simulink model "inversor_1"  (R2021b)
settings: Solver=FixedStepDiscrete  StartTime=0.0  StopTime=7  FixedStep=Tint  MaxStep=1e-6  RelTol=1e-6
InitFcn:
  | run init_fcn.m;
values from neighbouring files (symbols this model uses):
  C_load = 5e-2    (= 0.05)    [init_fcn.m]    (also in init_fcn_2.m)
  L_s = 5e-3    (= 0.005)    [init_fcn.m]    (also in init_fcn_2.m)
  R_load = 10    [init_fcn.m]    (also in init_fcn_2.m)
  shift = (180/2)/360 * Ts    (= 0.000125)    [init_fcn.m]    (also in init_fcn_2.m = 8.33333333333e-05)
  Tint = 1e-6    (= 1e-06)    [init_fcn.m]    (also in init_fcn_2.m)
  Ts = 1/2000    (= 0.0005)    [init_fcn.m]    (also in init_fcn_2.m)
  V_source = 230 * sqrt(2)    [init_fcn.m]    (also in init_fcn_2.m)
libraries: spsIGBTDiodeLib x8, spsVoltageMeasurementLib x6, simulink x3, spsSeriesRLCBranchLib x3, spsParallelRLCBranchLib x2, spsACVoltageSourceLib x1, spsCurrentMeasurementLib x1, spspowerguiLib x1
settings Model: Creator=david  LastModifiedBy=david

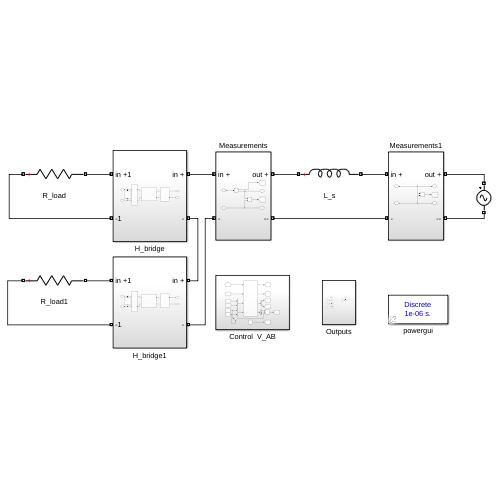
[thumbnail: Simulink's stored preview of the top-level diagram]
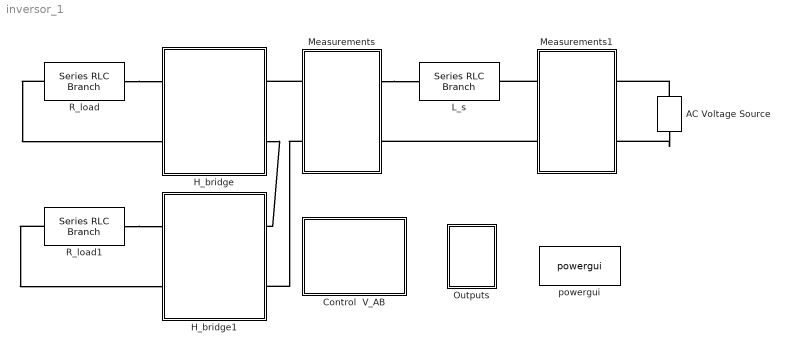
== system inversor_1 ==
  AC Voltage Source : spsACVoltageSourceLib/AC Voltage Source  Amplitude=V_source  Phase=0  Frequency=50  SampleTime=0  Measurements=None  BusType=swing  Pref=10e3  Qref=0  Qmin=-inf  Qmax=+inf
  Control  V_AB : Subsystem
  H_bridge : Subsystem
  H_bridge1 : Subsystem
  L_s : spsSeriesRLCBranchLib/Series RLC Branch  LConnTagsString=__new0  RConnTagsString=__new0  BranchType=L  Resistance=1  Inductance=L_s  SetiL0=off  InitialCurrent=0  Capacitance=1e-6  Setx0=off  InitialVoltage=0  Measurements=None
  Measurements : Subsystem
  Measurements1 : Subsystem
  Outputs : Subsystem
  R_load : spsSeriesRLCBranchLib/Series RLC Branch  LConnTagsString=__new0  RConnTagsString=__new0  BranchType=R  Resistance=R_load  Inductance=L_s  SetiL0=off  InitialCurrent=0  Capacitance=1e-6  Setx0=off  InitialVoltage=0  Measurements=None
  R_load1 : spsSeriesRLCBranchLib/Series RLC Branch  LConnTagsString=__new0  RConnTagsString=__new0  BranchType=R  Resistance=R_load  Inductance=L_s  SetiL0=off  InitialCurrent=0  Capacitance=1e-6  Setx0=off  InitialVoltage=0  Measurements=None
  powergui : spspowerguiLib/powergui  Priority=1  SimulationMode=Discrete  SampleTime=Tint  frequency=60  Iterations=50  frequencyindice=50  Pbase=100e6  ErrMax=1e-4  UnitsV=kV  UnitsW=MW  buscounter=0  FunctionMessages=off  echomessages=off  EnableUseOfTLC=off  CurrentSourceSwitches=off  DisableSnubberDevices=off  DisableRonSwitches=off  DisableVfSwitches=off  DisplayEquations=off  AutomaticDiscreteSolvers=off  SolverType=Tustin/Backward Euler (TBE)  Interpol=off  ExternalGateDelay=off  methode=off  Ts=100  x0status=blocks  SPID=on  SwTol=0  HookPort=off  NonlinearTolerance=1e-4  nMaxIteration=100  ContinueOnMaxIteration=off  RestoreLinks=warning  ResistiveCurrentMeasurement=off  Frange=[0:2:500]  Ylog=off  Xlog=on  ShowGrid=off  save=off  variable=ZData  structure=0  ZoomFFT=off  StartTime=0.0  cycles=1  DisplayStyle=1  fundamental=60  FreqAxis=off  MaxFrequency=1000  frequencyindicesteady=1  RmsSteady=1  display=off
  connections:
  R_load/LConn1 -- H_bridge/LConn2
  R_load/RConn1 -- H_bridge/LConn1
  Measurements/LConn1 -- H_bridge/RConn1
  Measurements/RConn1 -- L_s/LConn1
  Measurements1/LConn2 -- Measurements/RConn2
  Measurements1/LConn1 -- L_s/RConn1
  AC Voltage Source/RConn1 -- Measurements1/RConn1
  AC Voltage Source/LConn1 -- Measurements1/RConn2
  Measurements/LConn2 -- H_bridge1/RConn2
  R_load1/RConn1 -- H_bridge1/LConn1
  R_load1/LConn1 -- H_bridge1/LConn2
  H_bridge/RConn2 -- H_bridge1/RConn1

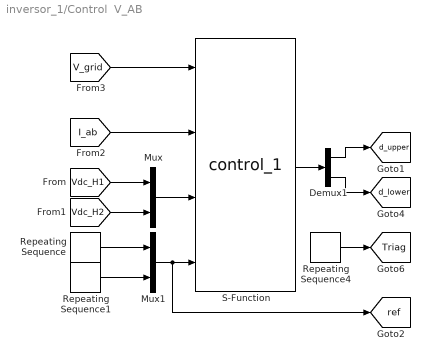
== system inversor_1/Control  V_AB ==
  Demux1 : Demux  Outputs=2
  Mux : Mux  Inputs=2
  Mux1 : Mux  Inputs=2
  Repeating Sequence : simulink/Sources/Repeating Sequence  rep_seq_t=[0 2 3 4 5 7]  rep_seq_y=[200 200 250 250 200 180]
  Repeating Sequence1 : simulink/Sources/Repeating Sequence  rep_seq_t=[0 2 3 4 5 7]  rep_seq_y=[200 200 150 150 230 230]
  Repeating Sequence4 : simulink/Sources/Repeating Sequence  rep_seq_t=[0 Ts/2 Ts]  rep_seq_y=[-1 1 -1]
  S-Function : S-Function  FunctionName=control_1  SFunctionDeploymentMode=off  EnableBusSupport=off
  tag scope: Triag=global, d_lower=global, d_upper=global, ref=global
  wires:
  Mux/1 -> S-Function/3
  [Vdc_H1] -> Mux/1
  [I_ab] -> S-Function/2
  [V_grid] -> S-Function/1
  Repeating Sequence/1 -> Mux1/1
  Repeating Sequence1/1 -> Mux1/2
  [Vdc_H2] -> Mux/2
  S-Function/1 -> Demux1/1
  Demux1/1 -> [d_upper]
  Demux1/2 -> [d_lower]
  Repeating Sequence4/1 -> [Triag]
  Mux1/1 -> [ref], S-Function/4

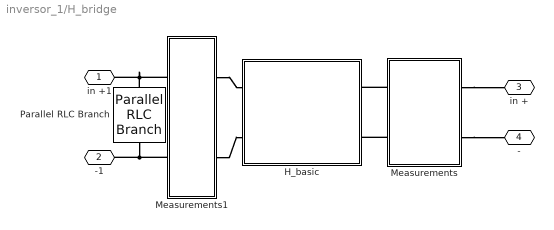
== system inversor_1/H_bridge ==
  H_basic : Subsystem
  Measurements : Subsystem
  Measurements1 : Subsystem
  Parallel RLC Branch : spsParallelRLCBranchLib/Parallel RLC Branch  LConnTagsString=a  RConnTagsString=__new0  BranchType=C  Resistance=1  Inductance=1e-3  SetiL0=off  InitialCurrent=0  Capacitance=C_load  Setx0=on  InitialVoltage=C_init_v  Measurements=None
  in +1 : PMIOPort  Side=Left
  -1 : PMIOPort  Port=2  Side=Left
  in + : PMIOPort  Port=3  Side=Right
  - : PMIOPort  Port=4  Side=Right
  connections:
  Measurements1/RConn1 -- H_basic/LConn1
  Measurements/LConn1 -- in +/RConn1
  Measurements1/RConn2 -- H_basic/LConn2
  Measurements1/LConn1 -- Parallel RLC Branch/LConn1 -- in +1/RConn1
  Measurements1/LConn2 -- Parallel RLC Branch/RConn1 -- -1/RConn1
  Measurements/RConn2 -- H_basic/RConn2
  Measurements/LConn2 -- -/RConn1
  Measurements/RConn1 -- H_basic/RConn1

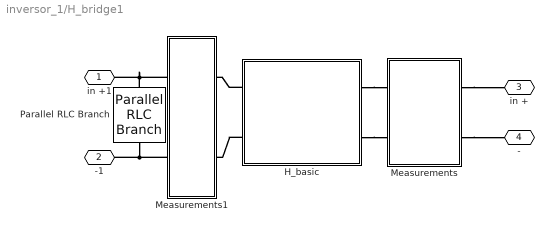
== system inversor_1/H_bridge1 ==
  H_basic : Subsystem
  Measurements : Subsystem
  Measurements1 : Subsystem
  Parallel RLC Branch : spsParallelRLCBranchLib/Parallel RLC Branch  LConnTagsString=a  RConnTagsString=__new0  BranchType=C  Resistance=1  Inductance=1e-3  SetiL0=off  InitialCurrent=0  Capacitance=C_load  Setx0=on  InitialVoltage=C_init_v  Measurements=None
  in +1 : PMIOPort  Side=Left
  -1 : PMIOPort  Port=2  Side=Left
  in + : PMIOPort  Port=3  Side=Right
  - : PMIOPort  Port=4  Side=Right
  connections:
  H_basic/LConn1 -- Measurements1/RConn1
  Measurements/LConn1 -- in +/RConn1
  H_basic/LConn2 -- Measurements1/RConn2
  Measurements1/LConn1 -- Parallel RLC Branch/LConn1 -- in +1/RConn1
  Measurements1/LConn2 -- Parallel RLC Branch/RConn1 -- -1/RConn1
  H_basic/RConn2 -- Measurements/RConn2
  Measurements/LConn2 -- -/RConn1
  H_basic/RConn1 -- Measurements/RConn1

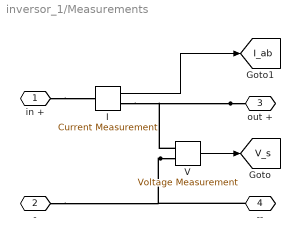
== system inversor_1/Measurements ==
  I : spsCurrentMeasurementLib/Current Measurement  PhasorSimulation=off  OutputType=Complex  PSBequivalent=0
  V : spsVoltageMeasurementLib/Voltage Measurement  PhasorSimulation=off  OutputType=Complex  PSBequivalent=0
  in + : PMIOPort  Side=Left
  - : PMIOPort  Port=2  Side=Left
  out + : PMIOPort  Port=3  Side=Right
  -- : PMIOPort  Port=4  Side=Right
  tag scope: I_ab=global, V_s=global
  wires:
  V/1 -> [V_s]
  I/1 -> [I_ab]
  connections:
  V/LConn2 -- --/RConn1 -- -/RConn1
  out +/RConn1 -- V/LConn1 -- I/RConn1
  in +/RConn1 -- I/LConn1

== system inversor_1/Measurements1 ==
  V : spsVoltageMeasurementLib/Voltage Measurement  PhasorSimulation=off  OutputType=Complex  PSBequivalent=0
  in + : PMIOPort  Side=Left
  - : PMIOPort  Port=2  Side=Left
  out + : PMIOPort  Port=3  Side=Right
  -- : PMIOPort  Port=4  Side=Right
  tag scope: V_grid=global
  wires:
  V/1 -> [V_grid]
  connections:
  V/LConn2 -- --/RConn1 -- -/RConn1
  out +/RConn1 -- in +/RConn1 -- V/LConn1

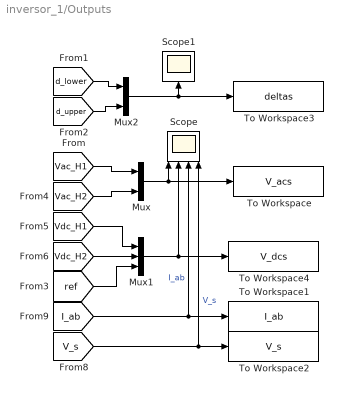
== system inversor_1/Outputs ==
  Mux : Mux  Inputs=2
  Mux1 : Mux  Inputs=3
  Mux2 : Mux  Inputs=2
  Scope : Scope  NumInputPorts=4
  Scope1 : Scope
  To Workspace : ToWorkspace  VariableName=V_acs  SaveFormat=Structure With Time  SampleTime=-1
  To Workspace1 : ToWorkspace  VariableName=I_ab  SaveFormat=Structure With Time  SampleTime=-1
  To Workspace2 : ToWorkspace  VariableName=V_s  SaveFormat=Structure With Time  SampleTime=-1
  To Workspace3 : ToWorkspace  VariableName=deltas  SaveFormat=Structure With Time  SampleTime=-1
  To Workspace4 : ToWorkspace  VariableName=V_dcs  SaveFormat=Structure With Time  SampleTime=-1
  wires:
  Mux/1 -> Scope/1, To Workspace/1
  [Vac_H1] -> Mux/1
  [Vac_H2] -> Mux/2
  Mux1/1 -> Scope/2, To Workspace4/1
  [V_s] -> Scope/4, To Workspace2/1  "V_s"
  [Vdc_H1] -> Mux1/1
  [Vdc_H2] -> Mux1/2
  [I_ab] -> Scope/3, To Workspace1/1  "I_ab"
  [d_lower] -> Mux2/1
  [d_upper] -> Mux2/2
  Mux2/1 -> Scope1/1, To Workspace3/1
  [ref] -> Mux1/3

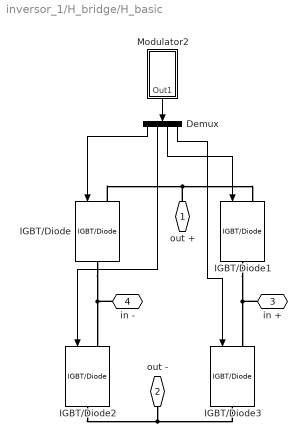
== system inversor_1/H_bridge/H_basic ==
  Demux : Demux
  IGBT/Diode{,1..3} (4 alike) : spsIGBTDiodeLib/IGBT//Diode  Ron=1e-3  Rs=1e5  Cs=inf  Measurements=off
  Modulator2 : Subsystem
  out + : PMIOPort  Side=Left
  out - : PMIOPort  Port=2  Side=Left
  in + : PMIOPort  Port=3  Side=Right
  in - : PMIOPort  Port=4  Side=Right
  wires:
  Demux/1 -> IGBT/Diode/1
  Demux/4 -> IGBT/Diode3/1
  Demux/2 -> IGBT/Diode2/1
  Demux/3 -> IGBT/Diode1/1
  Modulator2/1(Out1) -> Demux/1
  connections:
  IGBT/Diode2/RConn1 -- out -/RConn1 -- IGBT/Diode3/RConn1
  IGBT/Diode1/RConn1 -- in +/RConn1 -- IGBT/Diode3/LConn1
  IGBT/Diode/LConn1 -- out +/RConn1 -- IGBT/Diode1/LConn1
  IGBT/Diode/RConn1 -- in -/RConn1 -- IGBT/Diode2/LConn1

== system inversor_1/H_bridge/Measurements ==
  V : spsVoltageMeasurementLib/Voltage Measurement  PhasorSimulation=off  OutputType=Complex  PSBequivalent=0
  in + : PMIOPort  Side=Left
  - : PMIOPort  Port=2  Side=Left
  out + : PMIOPort  Port=3  Side=Right
  -- : PMIOPort  Port=4  Side=Right
  tag scope: Vac_H1=global
  wires:
  V/1 -> [Vac_H1]
  connections:
  V/LConn2 -- --/RConn1 -- -/RConn1
  V/LConn1 -- in +/RConn1 -- out +/RConn1

== system inversor_1/H_bridge/Measurements1 ==
  V : spsVoltageMeasurementLib/Voltage Measurement  PhasorSimulation=off  OutputType=Complex  PSBequivalent=0
  in + : PMIOPort  Side=Left
  - : PMIOPort  Port=2  Side=Left
  out + : PMIOPort  Port=3  Side=Right
  -- : PMIOPort  Port=4  Side=Right
  tag scope: Vdc_H1=global
  wires:
  V/1 -> [Vdc_H1]
  connections:
  -/RConn1 -- V/LConn2 -- --/RConn1
  V/LConn1 -- in +/RConn1 -- out +/RConn1

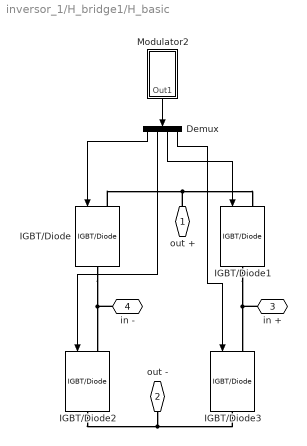
== system inversor_1/H_bridge1/H_basic ==
  Demux : Demux
  IGBT/Diode{,1..3} (4 alike) : spsIGBTDiodeLib/IGBT//Diode  Ron=1e-3  Rs=1e5  Cs=inf  Measurements=off
  Modulator2 : Subsystem
  out + : PMIOPort  Side=Left
  out - : PMIOPort  Port=2  Side=Left
  in + : PMIOPort  Port=3  Side=Right
  in - : PMIOPort  Port=4  Side=Right
  wires:
  Demux/1 -> IGBT/Diode/1
  Demux/4 -> IGBT/Diode3/1
  Demux/2 -> IGBT/Diode2/1
  Demux/3 -> IGBT/Diode1/1
  Modulator2/1(Out1) -> Demux/1
  connections:
  IGBT/Diode2/RConn1 -- out -/RConn1 -- IGBT/Diode3/RConn1
  IGBT/Diode1/RConn1 -- in +/RConn1 -- IGBT/Diode3/LConn1
  IGBT/Diode/LConn1 -- out +/RConn1 -- IGBT/Diode1/LConn1
  IGBT/Diode/RConn1 -- in -/RConn1 -- IGBT/Diode2/LConn1

== system inversor_1/H_bridge1/Measurements ==
  V : spsVoltageMeasurementLib/Voltage Measurement  PhasorSimulation=off  OutputType=Complex  PSBequivalent=0
  in + : PMIOPort  Side=Left
  - : PMIOPort  Port=2  Side=Left
  out + : PMIOPort  Port=3  Side=Right
  -- : PMIOPort  Port=4  Side=Right
  tag scope: Vac_H2=global
  wires:
  V/1 -> [Vac_H2]
  connections:
  V/LConn2 -- --/RConn1 -- -/RConn1
  V/LConn1 -- in +/RConn1 -- out +/RConn1

== system inversor_1/H_bridge1/Measurements1 ==
  V : spsVoltageMeasurementLib/Voltage Measurement  PhasorSimulation=off  OutputType=Complex  PSBequivalent=0
  in + : PMIOPort  Side=Left
  - : PMIOPort  Port=2  Side=Left
  out + : PMIOPort  Port=3  Side=Right
  -- : PMIOPort  Port=4  Side=Right
  tag scope: Vdc_H2=global
  wires:
  V/1 -> [Vdc_H2]
  connections:
  -/RConn1 -- V/LConn2 -- --/RConn1
  V/LConn1 -- in +/RConn1 -- out +/RConn1

== system inversor_1/H_bridge/H_basic/Modulator2 ==
  Mux : Mux
  Restriccion : Subsystem
  Unipolar : Subsystem
  Out1 : Outport
  wires:
  Restriccion/1(Out1) -> Mux/1
  [d_upper] -> Unipolar/1(Duty)
  Mux/1 -> Out1/1
  Restriccion/4(Out4) -> Mux/4
  Unipolar/1(Out1) -> Restriccion/1(In1)
  Restriccion/3(Out3) -> Mux/3
  Unipolar/2(Out2) -> Restriccion/2(In2)
  Restriccion/2(Out2) -> Mux/2
  [Triag] -> Unipolar/2(Triag)

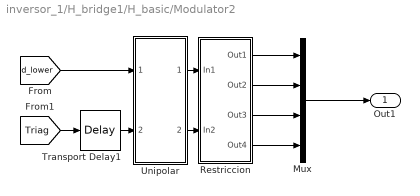
== system inversor_1/H_bridge1/H_basic/Modulator2 ==
  Mux : Mux
  Restriccion : Subsystem
  Transport Delay1 : TransportDelay  DelayTime=shift
  Unipolar : Subsystem
  Out1 : Outport
  wires:
  Restriccion/1(Out1) -> Mux/1
  [d_lower] -> Unipolar/1(Duty)
  Mux/1 -> Out1/1
  Restriccion/4(Out4) -> Mux/4
  Unipolar/1(Out1) -> Restriccion/1(In1)
  Restriccion/3(Out3) -> Mux/3
  Unipolar/2(Out2) -> Restriccion/2(In2)
  Restriccion/2(Out2) -> Mux/2
  [Triag] -> Transport Delay1/1
  Transport Delay1/1 -> Unipolar/2(Triag)

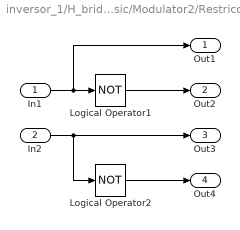
== system inversor_1/H_bridge/H_basic/Modulator2/Restriccion ==
  In1 : Inport
  In2 : Inport  Port=2
  Logical Operator1 : Logic  Operator=NOT  AllPortsSameDT=off  OutDataTypeStr=boolean
  Logical Operator2 : Logic  Operator=NOT  AllPortsSameDT=off  OutDataTypeStr=boolean
  Out1 : Outport
  Out2 : Outport  Port=2
  Out3 : Outport  Port=3
  Out4 : Outport  Port=4
  wires:
  In1/1 -> Out1/1, Logical Operator1/1
  In2/1 -> Out3/1, Logical Operator2/1
  Logical Operator2/1 -> Out4/1
  Logical Operator1/1 -> Out2/1

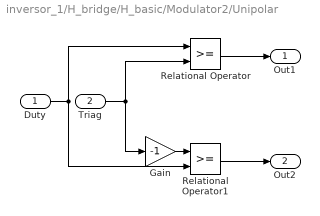
== system inversor_1/H_bridge/H_basic/Modulator2/Unipolar ==
  Duty : Inport
  Triag : Inport  Port=2
  Gain : Gain  Gain=-1
  Relational Operator : RelationalOperator  OutDataTypeStr=boolean  RndMeth=Simplest
  Relational Operator1 : RelationalOperator  OutDataTypeStr=boolean  RndMeth=Simplest
  Out1 : Outport
  Out2 : Outport  Port=2
  wires:
  Relational Operator/1 -> Out1/1
  Triag/1 -> Relational Operator/2, Gain/1
  Duty/1 -> Relational Operator1/2, Relational Operator/1
  Relational Operator1/1 -> Out2/1
  Gain/1 -> Relational Operator1/1

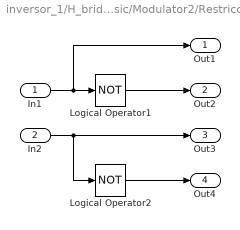
== system inversor_1/H_bridge1/H_basic/Modulator2/Restriccion ==
  In1 : Inport
  In2 : Inport  Port=2
  Logical Operator1 : Logic  Operator=NOT  AllPortsSameDT=off  OutDataTypeStr=boolean
  Logical Operator2 : Logic  Operator=NOT  AllPortsSameDT=off  OutDataTypeStr=boolean
  Out1 : Outport
  Out2 : Outport  Port=2
  Out3 : Outport  Port=3
  Out4 : Outport  Port=4
  wires:
  In1/1 -> Out1/1, Logical Operator1/1
  In2/1 -> Out3/1, Logical Operator2/1
  Logical Operator2/1 -> Out4/1
  Logical Operator1/1 -> Out2/1

== system inversor_1/H_bridge1/H_basic/Modulator2/Unipolar ==
  Duty : Inport
  Triag : Inport  Port=2
  Gain : Gain  Gain=-1
  Relational Operator : RelationalOperator  OutDataTypeStr=boolean  RndMeth=Simplest
  Relational Operator1 : RelationalOperator  OutDataTypeStr=boolean  RndMeth=Simplest
  Out1 : Outport
  Out2 : Outport  Port=2
  wires:
  Relational Operator/1 -> Out1/1
  Triag/1 -> Relational Operator/2, Gain/1
  Duty/1 -> Relational Operator1/2, Relational Operator/1
  Relational Operator1/1 -> Out2/1
  Gain/1 -> Relational Operator1/1
